simulink model "Architecture"  (R2020b)
settings: Solver=VariableStepAuto  StartTime=0.0  StopTime=10.0  RelTol=1e-3
undefined symbols (not defined in the file or in its folder): des, T
libraries: simulink x16
(part 4 of 6)

== system Architecture/PE11/Create Generator Selection Variable ==
  function : TriggerPort  TriggerType=function-call  VariantControl=(inherit)
  Repeating Sequence Stair : simulink/Sources/Repeating Sequence Stair  OutValues=[0 1].'  tsamp=-1  OutMin=[]  OutMax=[]  OutDataTypeStr=float('double')  OutputDataTypeScalingMode=Specify via dialog  OutDataType=float('double')  ConRadixGroup=Best Precision: Vector-wise  OutScaling=2^-12
  Out1 : Outport
  wires:
  Repeating Sequence Stair/1 -> Out1/1

== system Architecture/PE12/Create Generator Selection Variable ==
  function : TriggerPort  TriggerType=function-call  VariantControl=(inherit)
  Repeating Sequence Stair : simulink/Sources/Repeating Sequence Stair  OutValues=[0 1].'  tsamp=-1  OutMin=[]  OutMax=[]  OutDataTypeStr=float('double')  OutputDataTypeScalingMode=Specify via dialog  OutDataType=float('double')  ConRadixGroup=Best Precision: Vector-wise  OutScaling=2^-12
  Out1 : Outport
  wires:
  Repeating Sequence Stair/1 -> Out1/1

== system Architecture/PE13/Create Generator Selection Variable ==
  function : TriggerPort  TriggerType=function-call  VariantControl=(inherit)
  Repeating Sequence Stair : simulink/Sources/Repeating Sequence Stair  OutValues=[0 1].'  tsamp=-1  OutMin=[]  OutMax=[]  OutDataTypeStr=float('double')  OutputDataTypeScalingMode=Specify via dialog  OutDataType=float('double')  ConRadixGroup=Best Precision: Vector-wise  OutScaling=2^-12
  Out1 : Outport
  wires:
  Repeating Sequence Stair/1 -> Out1/1

== system Architecture/PE14/Create Generator Selection Variable ==
  function : TriggerPort  TriggerType=function-call  VariantControl=(inherit)
  Repeating Sequence Stair : simulink/Sources/Repeating Sequence Stair  OutValues=[0 1].'  tsamp=-1  OutMin=[]  OutMax=[]  OutDataTypeStr=float('double')  OutputDataTypeScalingMode=Specify via dialog  OutDataType=float('double')  ConRadixGroup=Best Precision: Vector-wise  OutScaling=2^-12
  Out1 : Outport
  wires:
  Repeating Sequence Stair/1 -> Out1/1

== system Architecture/PE15/Create Generator Selection Variable ==
  function : TriggerPort  TriggerType=function-call  VariantControl=(inherit)
  Repeating Sequence Stair : simulink/Sources/Repeating Sequence Stair  OutValues=[0 1].'  tsamp=-1  OutMin=[]  OutMax=[]  OutDataTypeStr=float('double')  OutputDataTypeScalingMode=Specify via dialog  OutDataType=float('double')  ConRadixGroup=Best Precision: Vector-wise  OutScaling=2^-12
  Out1 : Outport
  wires:
  Repeating Sequence Stair/1 -> Out1/1

== system Architecture/PE16/Create Generator Selection Variable ==
  function : TriggerPort  TriggerType=function-call  VariantControl=(inherit)
  Repeating Sequence Stair : simulink/Sources/Repeating Sequence Stair  OutValues=[0 1].'  tsamp=-1  OutMin=[]  OutMax=[]  OutDataTypeStr=float('double')  OutputDataTypeScalingMode=Specify via dialog  OutDataType=float('double')  ConRadixGroup=Best Precision: Vector-wise  OutScaling=2^-12
  Out1 : Outport
  wires:
  Repeating Sequence Stair/1 -> Out1/1

== system Architecture/PE2/Create Generator Selection Variable ==
  function : TriggerPort  TriggerType=function-call  VariantControl=(inherit)
  Repeating Sequence Stair : simulink/Sources/Repeating Sequence Stair  OutValues=[0 1].'  tsamp=-1  OutMin=[]  OutMax=[]  OutDataTypeStr=float('double')  OutputDataTypeScalingMode=Specify via dialog  OutDataType=float('double')  ConRadixGroup=Best Precision: Vector-wise  OutScaling=2^-12
  Out1 : Outport
  wires:
  Repeating Sequence Stair/1 -> Out1/1

== system Architecture/PE3/Create Generator Selection Variable ==
  function : TriggerPort  TriggerType=function-call  VariantControl=(inherit)
  Repeating Sequence Stair : simulink/Sources/Repeating Sequence Stair  OutValues=[0 1].'  tsamp=-1  OutMin=[]  OutMax=[]  OutDataTypeStr=float('double')  OutputDataTypeScalingMode=Specify via dialog  OutDataType=float('double')  ConRadixGroup=Best Precision: Vector-wise  OutScaling=2^-12
  Out1 : Outport
  wires:
  Repeating Sequence Stair/1 -> Out1/1

== system Architecture/PE4/Create Generator Selection Variable ==
  function : TriggerPort  TriggerType=function-call  VariantControl=(inherit)
  Repeating Sequence Stair : simulink/Sources/Repeating Sequence Stair  OutValues=[0 1].'  tsamp=-1  OutMin=[]  OutMax=[]  OutDataTypeStr=float('double')  OutputDataTypeScalingMode=Specify via dialog  OutDataType=float('double')  ConRadixGroup=Best Precision: Vector-wise  OutScaling=2^-12
  Out1 : Outport
  wires:
  Repeating Sequence Stair/1 -> Out1/1

== system Architecture/PE5/Create Generator Selection Variable ==
  function : TriggerPort  TriggerType=function-call  VariantControl=(inherit)
  Repeating Sequence Stair : simulink/Sources/Repeating Sequence Stair  OutValues=[0 1].'  tsamp=-1  OutMin=[]  OutMax=[]  OutDataTypeStr=float('double')  OutputDataTypeScalingMode=Specify via dialog  OutDataType=float('double')  ConRadixGroup=Best Precision: Vector-wise  OutScaling=2^-12
  Out1 : Outport
  wires:
  Repeating Sequence Stair/1 -> Out1/1

== system Architecture/PE6/Create Generator Selection Variable ==
  function : TriggerPort  TriggerType=function-call  VariantControl=(inherit)
  Repeating Sequence Stair : simulink/Sources/Repeating Sequence Stair  OutValues=[0 1].'  tsamp=-1  OutMin=[]  OutMax=[]  OutDataTypeStr=float('double')  OutputDataTypeScalingMode=Specify via dialog  OutDataType=float('double')  ConRadixGroup=Best Precision: Vector-wise  OutScaling=2^-12
  Out1 : Outport
  wires:
  Repeating Sequence Stair/1 -> Out1/1

== system Architecture/PE7/Create Generator Selection Variable ==
  function : TriggerPort  TriggerType=function-call  VariantControl=(inherit)
  Repeating Sequence Stair : simulink/Sources/Repeating Sequence Stair  OutValues=[0 1].'  tsamp=-1  OutMin=[]  OutMax=[]  OutDataTypeStr=float('double')  OutputDataTypeScalingMode=Specify via dialog  OutDataType=float('double')  ConRadixGroup=Best Precision: Vector-wise  OutScaling=2^-12
  Out1 : Outport
  wires:
  Repeating Sequence Stair/1 -> Out1/1

== system Architecture/PE8/Create Generator Selection Variable ==
  function : TriggerPort  TriggerType=function-call  VariantControl=(inherit)
  Repeating Sequence Stair : simulink/Sources/Repeating Sequence Stair  OutValues=[0 1].'  tsamp=-1  OutMin=[]  OutMax=[]  OutDataTypeStr=float('double')  OutputDataTypeScalingMode=Specify via dialog  OutDataType=float('double')  ConRadixGroup=Best Precision: Vector-wise  OutScaling=2^-12
  Out1 : Outport
  wires:
  Repeating Sequence Stair/1 -> Out1/1

== system Architecture/PE9/Create Generator Selection Variable ==
  function : TriggerPort  TriggerType=function-call  VariantControl=(inherit)
  Repeating Sequence Stair : simulink/Sources/Repeating Sequence Stair  OutValues=[0 1].'  tsamp=-1  OutMin=[]  OutMax=[]  OutDataTypeStr=float('double')  OutputDataTypeScalingMode=Specify via dialog  OutDataType=float('double')  ConRadixGroup=Best Precision: Vector-wise  OutScaling=2^-12
  Out1 : Outport
  wires:
  Repeating Sequence Stair/1 -> Out1/1

== system Architecture/Router1/Attribute Function ==
  MATLAB Function : MATLAB Function  TreatAsAtomicUnit=on
  __DMLF__EDE2FCE__ : EntityDepartureFunctionCallGenerator  TimingFunctionCallF1=Before entity departure  IsInsideAFB=on
  __DMLF__GA__ : GetAttribute  AttributeName=DST|ME  AttributeMissing=Error|Error  AttributeDefaultValue=1|1  AttributeTreatAsVector=1|1  AttributeSendTiming=Before entity departure|Before entity departure  EvaluatedDefaultAttributeValue={ [];[]}  IsInsideAFB=on
      settings: OutputPortMap=o1,o2
  __DMLF__SA__ : SetAttribute  AttributeName=RT  AttributeFrom=Signal port  EvaluatedAttributeValue={ []}  IsInsideAFB=on
  IN : PMIOPort  Side=Left
  OUT : PMIOPort  Port=2  Side=Right
  wires:
  MATLAB Function/1(out_RT) -> __DMLF__SA__/1
  __DMLF__GA__/2 -> MATLAB Function/2(ME)
  __DMLF__GA__/1 -> MATLAB Function/1(DST)
  __DMLF__EDE2FCE__/1 -> MATLAB Function/Trigger
  connections:
  __DMLF__SA__/RConn1 -- OUT/RConn1
  IN/RConn1 -- __DMLF__GA__/LConn1
  __DMLF__GA__/RConn1 -- __DMLF__EDE2FCE__/LConn1
  __DMLF__SA__/LConn1 -- __DMLF__EDE2FCE__/RConn1

== system Architecture/Router1/Clocked FIFO1 ==
  Event-Based Random Number : EventBasedRandomNumber  Distribution=Gaussian (normal)  meanNorm=E  stdNorm=S
  FIFO Queue : FIFOQueue  Capacity=F  StatNumberInBlock=on
      settings: OutputPortMap=o1
  Release Gate : ReleaseGate  OpenGateUpon=Function call from port fcn
  Time-Based Function-Call Generator : TimeBasedFunctionCallGenerator  EventGenerationMode=Period from port  Period=T
  Input : PMIOPort  Side=Left
  Output : PMIOPort  Port=2  Side=Right
  #n : Outport
  wires:
  Event-Based Random Number/1 -> Time-Based Function-Call Generator/1
  FIFO Queue/1 -> #n/1
  Time-Based Function-Call Generator/1 -> Release Gate/1
  connections:
  FIFO Queue/RConn1 -- Release Gate/LConn1
  Release Gate/RConn1 -- Output/RConn1
  FIFO Queue/LConn1 -- Input/RConn1

== system Architecture/Router1/Clocked FIFO2 ==
  Event-Based Random Number : EventBasedRandomNumber  Distribution=Gaussian (normal)  meanNorm=E  stdNorm=S
  FIFO Queue : FIFOQueue  Capacity=F  StatNumberInBlock=on
      settings: OutputPortMap=o1
  Release Gate : ReleaseGate  OpenGateUpon=Function call from port fcn
  Time-Based Function-Call Generator : TimeBasedFunctionCallGenerator  EventGenerationMode=Period from port  Period=T
  Input : PMIOPort  Side=Left
  Output : PMIOPort  Port=2  Side=Right
  #n : Outport
  wires:
  Event-Based Random Number/1 -> Time-Based Function-Call Generator/1
  FIFO Queue/1 -> #n/1
  Time-Based Function-Call Generator/1 -> Release Gate/1
  connections:
  FIFO Queue/RConn1 -- Release Gate/LConn1
  Release Gate/RConn1 -- Output/RConn1
  FIFO Queue/LConn1 -- Input/RConn1

== system Architecture/Router1/Clocked FIFO3 ==
  Event-Based Random Number : EventBasedRandomNumber  Distribution=Gaussian (normal)  meanNorm=E  stdNorm=S
  FIFO Queue : FIFOQueue  Capacity=F  StatNumberInBlock=on
      settings: OutputPortMap=o1
  Release Gate : ReleaseGate  OpenGateUpon=Function call from port fcn
  Time-Based Function-Call Generator : TimeBasedFunctionCallGenerator  EventGenerationMode=Period from port  Period=T
  Input : PMIOPort  Side=Left
  Output : PMIOPort  Port=2  Side=Right
  #n : Outport
  wires:
  Event-Based Random Number/1 -> Time-Based Function-Call Generator/1
  FIFO Queue/1 -> #n/1
  Time-Based Function-Call Generator/1 -> Release Gate/1
  connections:
  FIFO Queue/RConn1 -- Release Gate/LConn1
  Release Gate/RConn1 -- Output/RConn1
  FIFO Queue/LConn1 -- Input/RConn1

== system Architecture/Router1/Clocked FIFO4 ==
  Event-Based Random Number : EventBasedRandomNumber  Distribution=Gaussian (normal)  meanNorm=E  stdNorm=S
  FIFO Queue : FIFOQueue  Capacity=F  StatNumberInBlock=on
      settings: OutputPortMap=o1
  Release Gate : ReleaseGate  OpenGateUpon=Function call from port fcn
  Time-Based Function-Call Generator : TimeBasedFunctionCallGenerator  EventGenerationMode=Period from port  Period=T
  Input : PMIOPort  Side=Left
  Output : PMIOPort  Port=2  Side=Right
  #n : Outport
  wires:
  Event-Based Random Number/1 -> Time-Based Function-Call Generator/1
  FIFO Queue/1 -> #n/1
  Time-Based Function-Call Generator/1 -> Release Gate/1
  connections:
  FIFO Queue/RConn1 -- Release Gate/LConn1
  Release Gate/RConn1 -- Output/RConn1
  FIFO Queue/LConn1 -- Input/RConn1

== system Architecture/Router1/Clocked FIFO5 ==
  Event-Based Random Number : EventBasedRandomNumber  Distribution=Gaussian (normal)  meanNorm=E  stdNorm=S
  FIFO Queue : FIFOQueue  Capacity=F  StatNumberInBlock=on
      settings: OutputPortMap=o1
  Release Gate : ReleaseGate  OpenGateUpon=Function call from port fcn
  Time-Based Function-Call Generator : TimeBasedFunctionCallGenerator  EventGenerationMode=Period from port  Period=T
  Input : PMIOPort  Side=Left
  Output : PMIOPort  Port=2  Side=Right
  #n : Outport
  wires:
  Event-Based Random Number/1 -> Time-Based Function-Call Generator/1
  FIFO Queue/1 -> #n/1
  Time-Based Function-Call Generator/1 -> Release Gate/1
  connections:
  FIFO Queue/RConn1 -- Release Gate/LConn1
  Release Gate/RConn1 -- Output/RConn1
  FIFO Queue/LConn1 -- Input/RConn1

== system Architecture/Router10/Attribute Function ==
  MATLAB Function : MATLAB Function  TreatAsAtomicUnit=on
  __DMLF__EDE2FCE__ : EntityDepartureFunctionCallGenerator  TimingFunctionCallF1=Before entity departure  IsInsideAFB=on
  __DMLF__GA__ : GetAttribute  AttributeName=DST|ME  AttributeMissing=Error|Error  AttributeDefaultValue=1|1  AttributeTreatAsVector=1|1  AttributeSendTiming=Before entity departure|Before entity departure  EvaluatedDefaultAttributeValue={ [];[]}  IsInsideAFB=on
      settings: OutputPortMap=o1,o2
  __DMLF__SA__ : SetAttribute  AttributeName=RT  AttributeFrom=Signal port  EvaluatedAttributeValue={ []}  IsInsideAFB=on
  IN : PMIOPort  Side=Left
  OUT : PMIOPort  Port=2  Side=Right
  wires:
  MATLAB Function/1(out_RT) -> __DMLF__SA__/1
  __DMLF__GA__/2 -> MATLAB Function/2(ME)
  __DMLF__GA__/1 -> MATLAB Function/1(DST)
  __DMLF__EDE2FCE__/1 -> MATLAB Function/Trigger
  connections:
  __DMLF__SA__/RConn1 -- OUT/RConn1
  IN/RConn1 -- __DMLF__GA__/LConn1
  __DMLF__GA__/RConn1 -- __DMLF__EDE2FCE__/LConn1
  __DMLF__SA__/LConn1 -- __DMLF__EDE2FCE__/RConn1

== system Architecture/Router10/Clocked FIFO1 ==
  Event-Based Random Number : EventBasedRandomNumber  Distribution=Gaussian (normal)  meanNorm=E  stdNorm=S
  FIFO Queue : FIFOQueue  Capacity=F  StatNumberInBlock=on
      settings: OutputPortMap=o1
  Release Gate : ReleaseGate  OpenGateUpon=Function call from port fcn
  Time-Based Function-Call Generator : TimeBasedFunctionCallGenerator  EventGenerationMode=Period from port  Period=T
  Input : PMIOPort  Side=Left
  Output : PMIOPort  Port=2  Side=Right
  #n : Outport
  wires:
  Event-Based Random Number/1 -> Time-Based Function-Call Generator/1
  FIFO Queue/1 -> #n/1
  Time-Based Function-Call Generator/1 -> Release Gate/1
  connections:
  FIFO Queue/RConn1 -- Release Gate/LConn1
  Release Gate/RConn1 -- Output/RConn1
  FIFO Queue/LConn1 -- Input/RConn1

== system Architecture/Router10/Clocked FIFO2 ==
  Event-Based Random Number : EventBasedRandomNumber  Distribution=Gaussian (normal)  meanNorm=E  stdNorm=S
  FIFO Queue : FIFOQueue  Capacity=F  StatNumberInBlock=on
      settings: OutputPortMap=o1
  Release Gate : ReleaseGate  OpenGateUpon=Function call from port fcn
  Time-Based Function-Call Generator : TimeBasedFunctionCallGenerator  EventGenerationMode=Period from port  Period=T
  Input : PMIOPort  Side=Left
  Output : PMIOPort  Port=2  Side=Right
  #n : Outport
  wires:
  Event-Based Random Number/1 -> Time-Based Function-Call Generator/1
  FIFO Queue/1 -> #n/1
  Time-Based Function-Call Generator/1 -> Release Gate/1
  connections:
  FIFO Queue/RConn1 -- Release Gate/LConn1
  Release Gate/RConn1 -- Output/RConn1
  FIFO Queue/LConn1 -- Input/RConn1

== system Architecture/Router10/Clocked FIFO3 ==
  Event-Based Random Number : EventBasedRandomNumber  Distribution=Gaussian (normal)  meanNorm=E  stdNorm=S
  FIFO Queue : FIFOQueue  Capacity=F  StatNumberInBlock=on
      settings: OutputPortMap=o1
  Release Gate : ReleaseGate  OpenGateUpon=Function call from port fcn
  Time-Based Function-Call Generator : TimeBasedFunctionCallGenerator  EventGenerationMode=Period from port  Period=T
  Input : PMIOPort  Side=Left
  Output : PMIOPort  Port=2  Side=Right
  #n : Outport
  wires:
  Event-Based Random Number/1 -> Time-Based Function-Call Generator/1
  FIFO Queue/1 -> #n/1
  Time-Based Function-Call Generator/1 -> Release Gate/1
  connections:
  FIFO Queue/RConn1 -- Release Gate/LConn1
  Release Gate/RConn1 -- Output/RConn1
  FIFO Queue/LConn1 -- Input/RConn1

== system Architecture/Router10/Clocked FIFO4 ==
  Event-Based Random Number : EventBasedRandomNumber  Distribution=Gaussian (normal)  meanNorm=E  stdNorm=S
  FIFO Queue : FIFOQueue  Capacity=F  StatNumberInBlock=on
      settings: OutputPortMap=o1
  Release Gate : ReleaseGate  OpenGateUpon=Function call from port fcn
  Time-Based Function-Call Generator : TimeBasedFunctionCallGenerator  EventGenerationMode=Period from port  Period=T
  Input : PMIOPort  Side=Left
  Output : PMIOPort  Port=2  Side=Right
  #n : Outport
  wires:
  Event-Based Random Number/1 -> Time-Based Function-Call Generator/1
  FIFO Queue/1 -> #n/1
  Time-Based Function-Call Generator/1 -> Release Gate/1
  connections:
  FIFO Queue/RConn1 -- Release Gate/LConn1
  Release Gate/RConn1 -- Output/RConn1
  FIFO Queue/LConn1 -- Input/RConn1

== system Architecture/Router10/Clocked FIFO5 ==
  Event-Based Random Number : EventBasedRandomNumber  Distribution=Gaussian (normal)  meanNorm=E  stdNorm=S
  FIFO Queue : FIFOQueue  Capacity=F  StatNumberInBlock=on
      settings: OutputPortMap=o1
  Release Gate : ReleaseGate  OpenGateUpon=Function call from port fcn
  Time-Based Function-Call Generator : TimeBasedFunctionCallGenerator  EventGenerationMode=Period from port  Period=T
  Input : PMIOPort  Side=Left
  Output : PMIOPort  Port=2  Side=Right
  #n : Outport
  wires:
  Event-Based Random Number/1 -> Time-Based Function-Call Generator/1
  FIFO Queue/1 -> #n/1
  Time-Based Function-Call Generator/1 -> Release Gate/1
  connections:
  FIFO Queue/RConn1 -- Release Gate/LConn1
  Release Gate/RConn1 -- Output/RConn1
  FIFO Queue/LConn1 -- Input/RConn1

== system Architecture/Router11/Attribute Function ==
  MATLAB Function : MATLAB Function  TreatAsAtomicUnit=on
  __DMLF__EDE2FCE__ : EntityDepartureFunctionCallGenerator  TimingFunctionCallF1=Before entity departure  IsInsideAFB=on
  __DMLF__GA__ : GetAttribute  AttributeName=DST|ME  AttributeMissing=Error|Error  AttributeDefaultValue=1|1  AttributeTreatAsVector=1|1  AttributeSendTiming=Before entity departure|Before entity departure  EvaluatedDefaultAttributeValue={ [];[]}  IsInsideAFB=on
      settings: OutputPortMap=o1,o2
  __DMLF__SA__ : SetAttribute  AttributeName=RT  AttributeFrom=Signal port  EvaluatedAttributeValue={ []}  IsInsideAFB=on
  IN : PMIOPort  Side=Left
  OUT : PMIOPort  Port=2  Side=Right
  wires:
  MATLAB Function/1(out_RT) -> __DMLF__SA__/1
  __DMLF__GA__/2 -> MATLAB Function/2(ME)
  __DMLF__GA__/1 -> MATLAB Function/1(DST)
  __DMLF__EDE2FCE__/1 -> MATLAB Function/Trigger
  connections:
  __DMLF__SA__/RConn1 -- OUT/RConn1
  IN/RConn1 -- __DMLF__GA__/LConn1
  __DMLF__GA__/RConn1 -- __DMLF__EDE2FCE__/LConn1
  __DMLF__SA__/LConn1 -- __DMLF__EDE2FCE__/RConn1

== system Architecture/Router11/Clocked FIFO1 ==
  Event-Based Random Number : EventBasedRandomNumber  Distribution=Gaussian (normal)  meanNorm=E  stdNorm=S
  FIFO Queue : FIFOQueue  Capacity=F  StatNumberInBlock=on
      settings: OutputPortMap=o1
  Release Gate : ReleaseGate  OpenGateUpon=Function call from port fcn
  Time-Based Function-Call Generator : TimeBasedFunctionCallGenerator  EventGenerationMode=Period from port  Period=T
  Input : PMIOPort  Side=Left
  Output : PMIOPort  Port=2  Side=Right
  #n : Outport
  wires:
  Event-Based Random Number/1 -> Time-Based Function-Call Generator/1
  FIFO Queue/1 -> #n/1
  Time-Based Function-Call Generator/1 -> Release Gate/1
  connections:
  FIFO Queue/RConn1 -- Release Gate/LConn1
  Release Gate/RConn1 -- Output/RConn1
  FIFO Queue/LConn1 -- Input/RConn1

== system Architecture/Router11/Clocked FIFO2 ==
  Event-Based Random Number : EventBasedRandomNumber  Distribution=Gaussian (normal)  meanNorm=E  stdNorm=S
  FIFO Queue : FIFOQueue  Capacity=F  StatNumberInBlock=on
      settings: OutputPortMap=o1
  Release Gate : ReleaseGate  OpenGateUpon=Function call from port fcn
  Time-Based Function-Call Generator : TimeBasedFunctionCallGenerator  EventGenerationMode=Period from port  Period=T
  Input : PMIOPort  Side=Left
  Output : PMIOPort  Port=2  Side=Right
  #n : Outport
  wires:
  Event-Based Random Number/1 -> Time-Based Function-Call Generator/1
  FIFO Queue/1 -> #n/1
  Time-Based Function-Call Generator/1 -> Release Gate/1
  connections:
  FIFO Queue/RConn1 -- Release Gate/LConn1
  Release Gate/RConn1 -- Output/RConn1
  FIFO Queue/LConn1 -- Input/RConn1

== system Architecture/Router11/Clocked FIFO3 ==
  Event-Based Random Number : EventBasedRandomNumber  Distribution=Gaussian (normal)  meanNorm=E  stdNorm=S
  FIFO Queue : FIFOQueue  Capacity=F  StatNumberInBlock=on
      settings: OutputPortMap=o1
  Release Gate : ReleaseGate  OpenGateUpon=Function call from port fcn
  Time-Based Function-Call Generator : TimeBasedFunctionCallGenerator  EventGenerationMode=Period from port  Period=T
  Input : PMIOPort  Side=Left
  Output : PMIOPort  Port=2  Side=Right
  #n : Outport
  wires:
  Event-Based Random Number/1 -> Time-Based Function-Call Generator/1
  FIFO Queue/1 -> #n/1
  Time-Based Function-Call Generator/1 -> Release Gate/1
  connections:
  FIFO Queue/RConn1 -- Release Gate/LConn1
  Release Gate/RConn1 -- Output/RConn1
  FIFO Queue/LConn1 -- Input/RConn1

== system Architecture/Router11/Clocked FIFO4 ==
  Event-Based Random Number : EventBasedRandomNumber  Distribution=Gaussian (normal)  meanNorm=E  stdNorm=S
  FIFO Queue : FIFOQueue  Capacity=F  StatNumberInBlock=on
      settings: OutputPortMap=o1
  Release Gate : ReleaseGate  OpenGateUpon=Function call from port fcn
  Time-Based Function-Call Generator : TimeBasedFunctionCallGenerator  EventGenerationMode=Period from port  Period=T
  Input : PMIOPort  Side=Left
  Output : PMIOPort  Port=2  Side=Right
  #n : Outport
  wires:
  Event-Based Random Number/1 -> Time-Based Function-Call Generator/1
  FIFO Queue/1 -> #n/1
  Time-Based Function-Call Generator/1 -> Release Gate/1
  connections:
  FIFO Queue/RConn1 -- Release Gate/LConn1
  Release Gate/RConn1 -- Output/RConn1
  FIFO Queue/LConn1 -- Input/RConn1

== system Architecture/Router11/Clocked FIFO5 ==
  Event-Based Random Number : EventBasedRandomNumber  Distribution=Gaussian (normal)  meanNorm=E  stdNorm=S
  FIFO Queue : FIFOQueue  Capacity=F  StatNumberInBlock=on
      settings: OutputPortMap=o1
  Release Gate : ReleaseGate  OpenGateUpon=Function call from port fcn
  Time-Based Function-Call Generator : TimeBasedFunctionCallGenerator  EventGenerationMode=Period from port  Period=T
  Input : PMIOPort  Side=Left
  Output : PMIOPort  Port=2  Side=Right
  #n : Outport
  wires:
  Event-Based Random Number/1 -> Time-Based Function-Call Generator/1
  FIFO Queue/1 -> #n/1
  Time-Based Function-Call Generator/1 -> Release Gate/1
  connections:
  FIFO Queue/RConn1 -- Release Gate/LConn1
  Release Gate/RConn1 -- Output/RConn1
  FIFO Queue/LConn1 -- Input/RConn1

== system Architecture/Router12/Attribute Function ==
  MATLAB Function : MATLAB Function  TreatAsAtomicUnit=on
  __DMLF__EDE2FCE__ : EntityDepartureFunctionCallGenerator  TimingFunctionCallF1=Before entity departure  IsInsideAFB=on
  __DMLF__GA__ : GetAttribute  AttributeName=DST|ME  AttributeMissing=Error|Error  AttributeDefaultValue=1|1  AttributeTreatAsVector=1|1  AttributeSendTiming=Before entity departure|Before entity departure  EvaluatedDefaultAttributeValue={ [];[]}  IsInsideAFB=on
      settings: OutputPortMap=o1,o2
  __DMLF__SA__ : SetAttribute  AttributeName=RT  AttributeFrom=Signal port  EvaluatedAttributeValue={ []}  IsInsideAFB=on
  IN : PMIOPort  Side=Left
  OUT : PMIOPort  Port=2  Side=Right
  wires:
  MATLAB Function/1(out_RT) -> __DMLF__SA__/1
  __DMLF__GA__/2 -> MATLAB Function/2(ME)
  __DMLF__GA__/1 -> MATLAB Function/1(DST)
  __DMLF__EDE2FCE__/1 -> MATLAB Function/Trigger
  connections:
  __DMLF__SA__/RConn1 -- OUT/RConn1
  IN/RConn1 -- __DMLF__GA__/LConn1
  __DMLF__GA__/RConn1 -- __DMLF__EDE2FCE__/LConn1
  __DMLF__SA__/LConn1 -- __DMLF__EDE2FCE__/RConn1

== system Architecture/Router12/Clocked FIFO1 ==
  Event-Based Random Number : EventBasedRandomNumber  Distribution=Gaussian (normal)  meanNorm=E  stdNorm=S
  FIFO Queue : FIFOQueue  Capacity=F  StatNumberInBlock=on
      settings: OutputPortMap=o1
  Release Gate : ReleaseGate  OpenGateUpon=Function call from port fcn
  Time-Based Function-Call Generator : TimeBasedFunctionCallGenerator  EventGenerationMode=Period from port  Period=T
  Input : PMIOPort  Side=Left
  Output : PMIOPort  Port=2  Side=Right
  #n : Outport
  wires:
  Event-Based Random Number/1 -> Time-Based Function-Call Generator/1
  FIFO Queue/1 -> #n/1
  Time-Based Function-Call Generator/1 -> Release Gate/1
  connections:
  FIFO Queue/RConn1 -- Release Gate/LConn1
  Release Gate/RConn1 -- Output/RConn1
  FIFO Queue/LConn1 -- Input/RConn1

== system Architecture/Router12/Clocked FIFO2 ==
  Event-Based Random Number : EventBasedRandomNumber  Distribution=Gaussian (normal)  meanNorm=E  stdNorm=S
  FIFO Queue : FIFOQueue  Capacity=F  StatNumberInBlock=on
      settings: OutputPortMap=o1
  Release Gate : ReleaseGate  OpenGateUpon=Function call from port fcn
  Time-Based Function-Call Generator : TimeBasedFunctionCallGenerator  EventGenerationMode=Period from port  Period=T
  Input : PMIOPort  Side=Left
  Output : PMIOPort  Port=2  Side=Right
  #n : Outport
  wires:
  Event-Based Random Number/1 -> Time-Based Function-Call Generator/1
  FIFO Queue/1 -> #n/1
  Time-Based Function-Call Generator/1 -> Release Gate/1
  connections:
  FIFO Queue/RConn1 -- Release Gate/LConn1
  Release Gate/RConn1 -- Output/RConn1
  FIFO Queue/LConn1 -- Input/RConn1

== system Architecture/Router12/Clocked FIFO3 ==
  Event-Based Random Number : EventBasedRandomNumber  Distribution=Gaussian (normal)  meanNorm=E  stdNorm=S
  FIFO Queue : FIFOQueue  Capacity=F  StatNumberInBlock=on
      settings: OutputPortMap=o1
  Release Gate : ReleaseGate  OpenGateUpon=Function call from port fcn
  Time-Based Function-Call Generator : TimeBasedFunctionCallGenerator  EventGenerationMode=Period from port  Period=T
  Input : PMIOPort  Side=Left
  Output : PMIOPort  Port=2  Side=Right
  #n : Outport
  wires:
  Event-Based Random Number/1 -> Time-Based Function-Call Generator/1
  FIFO Queue/1 -> #n/1
  Time-Based Function-Call Generator/1 -> Release Gate/1
  connections:
  FIFO Queue/RConn1 -- Release Gate/LConn1
  Release Gate/RConn1 -- Output/RConn1
  FIFO Queue/LConn1 -- Input/RConn1

== system Architecture/Router12/Clocked FIFO4 ==
  Event-Based Random Number : EventBasedRandomNumber  Distribution=Gaussian (normal)  meanNorm=E  stdNorm=S
  FIFO Queue : FIFOQueue  Capacity=F  StatNumberInBlock=on
      settings: OutputPortMap=o1
  Release Gate : ReleaseGate  OpenGateUpon=Function call from port fcn
  Time-Based Function-Call Generator : TimeBasedFunctionCallGenerator  EventGenerationMode=Period from port  Period=T
  Input : PMIOPort  Side=Left
  Output : PMIOPort  Port=2  Side=Right
  #n : Outport
  wires:
  Event-Based Random Number/1 -> Time-Based Function-Call Generator/1
  FIFO Queue/1 -> #n/1
  Time-Based Function-Call Generator/1 -> Release Gate/1
  connections:
  FIFO Queue/RConn1 -- Release Gate/LConn1
  Release Gate/RConn1 -- Output/RConn1
  FIFO Queue/LConn1 -- Input/RConn1

== system Architecture/Router12/Clocked FIFO5 ==
  Event-Based Random Number : EventBasedRandomNumber  Distribution=Gaussian (normal)  meanNorm=E  stdNorm=S
  FIFO Queue : FIFOQueue  Capacity=F  StatNumberInBlock=on
      settings: OutputPortMap=o1
  Release Gate : ReleaseGate  OpenGateUpon=Function call from port fcn
  Time-Based Function-Call Generator : TimeBasedFunctionCallGenerator  EventGenerationMode=Period from port  Period=T
  Input : PMIOPort  Side=Left
  Output : PMIOPort  Port=2  Side=Right
  #n : Outport
  wires:
  Event-Based Random Number/1 -> Time-Based Function-Call Generator/1
  FIFO Queue/1 -> #n/1
  Time-Based Function-Call Generator/1 -> Release Gate/1
  connections:
  FIFO Queue/RConn1 -- Release Gate/LConn1
  Release Gate/RConn1 -- Output/RConn1
  FIFO Queue/LConn1 -- Input/RConn1

== system Architecture/Router13/Attribute Function ==
  MATLAB Function : MATLAB Function  TreatAsAtomicUnit=on
  __DMLF__EDE2FCE__ : EntityDepartureFunctionCallGenerator  TimingFunctionCallF1=Before entity departure  IsInsideAFB=on
  __DMLF__GA__ : GetAttribute  AttributeName=DST|ME  AttributeMissing=Error|Error  AttributeDefaultValue=1|1  AttributeTreatAsVector=1|1  AttributeSendTiming=Before entity departure|Before entity departure  EvaluatedDefaultAttributeValue={ [];[]}  IsInsideAFB=on
      settings: OutputPortMap=o1,o2
  __DMLF__SA__ : SetAttribute  AttributeName=RT  AttributeFrom=Signal port  EvaluatedAttributeValue={ []}  IsInsideAFB=on
  IN : PMIOPort  Side=Left
  OUT : PMIOPort  Port=2  Side=Right
  wires:
  MATLAB Function/1(out_RT) -> __DMLF__SA__/1
  __DMLF__GA__/2 -> MATLAB Function/2(ME)
  __DMLF__GA__/1 -> MATLAB Function/1(DST)
  __DMLF__EDE2FCE__/1 -> MATLAB Function/Trigger
  connections:
  __DMLF__SA__/RConn1 -- OUT/RConn1
  IN/RConn1 -- __DMLF__GA__/LConn1
  __DMLF__GA__/RConn1 -- __DMLF__EDE2FCE__/LConn1
  __DMLF__SA__/LConn1 -- __DMLF__EDE2FCE__/RConn1

== system Architecture/Router13/Clocked FIFO1 ==
  Event-Based Random Number : EventBasedRandomNumber  Distribution=Gaussian (normal)  meanNorm=E  stdNorm=S
  FIFO Queue : FIFOQueue  Capacity=F  StatNumberInBlock=on
      settings: OutputPortMap=o1
  Release Gate : ReleaseGate  OpenGateUpon=Function call from port fcn
  Time-Based Function-Call Generator : TimeBasedFunctionCallGenerator  EventGenerationMode=Period from port  Period=T
  Input : PMIOPort  Side=Left
  Output : PMIOPort  Port=2  Side=Right
  #n : Outport
  wires:
  Event-Based Random Number/1 -> Time-Based Function-Call Generator/1
  FIFO Queue/1 -> #n/1
  Time-Based Function-Call Generator/1 -> Release Gate/1
  connections:
  FIFO Queue/RConn1 -- Release Gate/LConn1
  Release Gate/RConn1 -- Output/RConn1
  FIFO Queue/LConn1 -- Input/RConn1

== system Architecture/Router13/Clocked FIFO2 ==
  Event-Based Random Number : EventBasedRandomNumber  Distribution=Gaussian (normal)  meanNorm=E  stdNorm=S
  FIFO Queue : FIFOQueue  Capacity=F  StatNumberInBlock=on
      settings: OutputPortMap=o1
  Release Gate : ReleaseGate  OpenGateUpon=Function call from port fcn
  Time-Based Function-Call Generator : TimeBasedFunctionCallGenerator  EventGenerationMode=Period from port  Period=T
  Input : PMIOPort  Side=Left
  Output : PMIOPort  Port=2  Side=Right
  #n : Outport
  wires:
  Event-Based Random Number/1 -> Time-Based Function-Call Generator/1
  FIFO Queue/1 -> #n/1
  Time-Based Function-Call Generator/1 -> Release Gate/1
  connections:
  FIFO Queue/RConn1 -- Release Gate/LConn1
  Release Gate/RConn1 -- Output/RConn1
  FIFO Queue/LConn1 -- Input/RConn1

== system Architecture/Router13/Clocked FIFO3 ==
  Event-Based Random Number : EventBasedRandomNumber  Distribution=Gaussian (normal)  meanNorm=E  stdNorm=S
  FIFO Queue : FIFOQueue  Capacity=F  StatNumberInBlock=on
      settings: OutputPortMap=o1
  Release Gate : ReleaseGate  OpenGateUpon=Function call from port fcn
  Time-Based Function-Call Generator : TimeBasedFunctionCallGenerator  EventGenerationMode=Period from port  Period=T
  Input : PMIOPort  Side=Left
  Output : PMIOPort  Port=2  Side=Right
  #n : Outport
  wires:
  Event-Based Random Number/1 -> Time-Based Function-Call Generator/1
  FIFO Queue/1 -> #n/1
  Time-Based Function-Call Generator/1 -> Release Gate/1
  connections:
  FIFO Queue/RConn1 -- Release Gate/LConn1
  Release Gate/RConn1 -- Output/RConn1
  FIFO Queue/LConn1 -- Input/RConn1

== system Architecture/Router13/Clocked FIFO4 ==
  Event-Based Random Number : EventBasedRandomNumber  Distribution=Gaussian (normal)  meanNorm=E  stdNorm=S
  FIFO Queue : FIFOQueue  Capacity=F  StatNumberInBlock=on
      settings: OutputPortMap=o1
  Release Gate : ReleaseGate  OpenGateUpon=Function call from port fcn
  Time-Based Function-Call Generator : TimeBasedFunctionCallGenerator  EventGenerationMode=Period from port  Period=T
  Input : PMIOPort  Side=Left
  Output : PMIOPort  Port=2  Side=Right
  #n : Outport
  wires:
  Event-Based Random Number/1 -> Time-Based Function-Call Generator/1
  FIFO Queue/1 -> #n/1
  Time-Based Function-Call Generator/1 -> Release Gate/1
  connections:
  FIFO Queue/RConn1 -- Release Gate/LConn1
  Release Gate/RConn1 -- Output/RConn1
  FIFO Queue/LConn1 -- Input/RConn1

== system Architecture/Router13/Clocked FIFO5 ==
  Event-Based Random Number : EventBasedRandomNumber  Distribution=Gaussian (normal)  meanNorm=E  stdNorm=S
  FIFO Queue : FIFOQueue  Capacity=F  StatNumberInBlock=on
      settings: OutputPortMap=o1
  Release Gate : ReleaseGate  OpenGateUpon=Function call from port fcn
  Time-Based Function-Call Generator : TimeBasedFunctionCallGenerator  EventGenerationMode=Period from port  Period=T
  Input : PMIOPort  Side=Left
  Output : PMIOPort  Port=2  Side=Right
  #n : Outport
  wires:
  Event-Based Random Number/1 -> Time-Based Function-Call Generator/1
  FIFO Queue/1 -> #n/1
  Time-Based Function-Call Generator/1 -> Release Gate/1
  connections:
  FIFO Queue/RConn1 -- Release Gate/LConn1
  Release Gate/RConn1 -- Output/RConn1
  FIFO Queue/LConn1 -- Input/RConn1

== system Architecture/Router14/Attribute Function ==
  MATLAB Function : MATLAB Function  TreatAsAtomicUnit=on
  __DMLF__EDE2FCE__ : EntityDepartureFunctionCallGenerator  TimingFunctionCallF1=Before entity departure  IsInsideAFB=on
  __DMLF__GA__ : GetAttribute  AttributeName=DST|ME  AttributeMissing=Error|Error  AttributeDefaultValue=1|1  AttributeTreatAsVector=1|1  AttributeSendTiming=Before entity departure|Before entity departure  EvaluatedDefaultAttributeValue={ [];[]}  IsInsideAFB=on
      settings: OutputPortMap=o1,o2
  __DMLF__SA__ : SetAttribute  AttributeName=RT  AttributeFrom=Signal port  EvaluatedAttributeValue={ []}  IsInsideAFB=on
  IN : PMIOPort  Side=Left
  OUT : PMIOPort  Port=2  Side=Right
  wires:
  MATLAB Function/1(out_RT) -> __DMLF__SA__/1
  __DMLF__GA__/2 -> MATLAB Function/2(ME)
  __DMLF__GA__/1 -> MATLAB Function/1(DST)
  __DMLF__EDE2FCE__/1 -> MATLAB Function/Trigger
  connections:
  __DMLF__SA__/RConn1 -- OUT/RConn1
  IN/RConn1 -- __DMLF__GA__/LConn1
  __DMLF__GA__/RConn1 -- __DMLF__EDE2FCE__/LConn1
  __DMLF__SA__/LConn1 -- __DMLF__EDE2FCE__/RConn1

== system Architecture/Router14/Clocked FIFO1 ==
  Event-Based Random Number : EventBasedRandomNumber  Distribution=Gaussian (normal)  meanNorm=E  stdNorm=S
  FIFO Queue : FIFOQueue  Capacity=F  StatNumberInBlock=on
      settings: OutputPortMap=o1
  Release Gate : ReleaseGate  OpenGateUpon=Function call from port fcn
  Time-Based Function-Call Generator : TimeBasedFunctionCallGenerator  EventGenerationMode=Period from port  Period=T
  Input : PMIOPort  Side=Left
  Output : PMIOPort  Port=2  Side=Right
  #n : Outport
  wires:
  Event-Based Random Number/1 -> Time-Based Function-Call Generator/1
  FIFO Queue/1 -> #n/1
  Time-Based Function-Call Generator/1 -> Release Gate/1
  connections:
  FIFO Queue/RConn1 -- Release Gate/LConn1
  Release Gate/RConn1 -- Output/RConn1
  FIFO Queue/LConn1 -- Input/RConn1

== system Architecture/Router14/Clocked FIFO2 ==
  Event-Based Random Number : EventBasedRandomNumber  Distribution=Gaussian (normal)  meanNorm=E  stdNorm=S
  FIFO Queue : FIFOQueue  Capacity=F  StatNumberInBlock=on
      settings: OutputPortMap=o1
  Release Gate : ReleaseGate  OpenGateUpon=Function call from port fcn
  Time-Based Function-Call Generator : TimeBasedFunctionCallGenerator  EventGenerationMode=Period from port  Period=T
  Input : PMIOPort  Side=Left
  Output : PMIOPort  Port=2  Side=Right
  #n : Outport
  wires:
  Event-Based Random Number/1 -> Time-Based Function-Call Generator/1
  FIFO Queue/1 -> #n/1
  Time-Based Function-Call Generator/1 -> Release Gate/1
  connections:
  FIFO Queue/RConn1 -- Release Gate/LConn1
  Release Gate/RConn1 -- Output/RConn1
  FIFO Queue/LConn1 -- Input/RConn1

== system Architecture/Router14/Clocked FIFO3 ==
  Event-Based Random Number : EventBasedRandomNumber  Distribution=Gaussian (normal)  meanNorm=E  stdNorm=S
  FIFO Queue : FIFOQueue  Capacity=F  StatNumberInBlock=on
      settings: OutputPortMap=o1
  Release Gate : ReleaseGate  OpenGateUpon=Function call from port fcn
  Time-Based Function-Call Generator : TimeBasedFunctionCallGenerator  EventGenerationMode=Period from port  Period=T
  Input : PMIOPort  Side=Left
  Output : PMIOPort  Port=2  Side=Right
  #n : Outport
  wires:
  Event-Based Random Number/1 -> Time-Based Function-Call Generator/1
  FIFO Queue/1 -> #n/1
  Time-Based Function-Call Generator/1 -> Release Gate/1
  connections:
  FIFO Queue/RConn1 -- Release Gate/LConn1
  Release Gate/RConn1 -- Output/RConn1
  FIFO Queue/LConn1 -- Input/RConn1

== system Architecture/Router14/Clocked FIFO4 ==
  Event-Based Random Number : EventBasedRandomNumber  Distribution=Gaussian (normal)  meanNorm=E  stdNorm=S
  FIFO Queue : FIFOQueue  Capacity=F  StatNumberInBlock=on
      settings: OutputPortMap=o1
  Release Gate : ReleaseGate  OpenGateUpon=Function call from port fcn
  Time-Based Function-Call Generator : TimeBasedFunctionCallGenerator  EventGenerationMode=Period from port  Period=T
  Input : PMIOPort  Side=Left
  Output : PMIOPort  Port=2  Side=Right
  #n : Outport
  wires:
  Event-Based Random Number/1 -> Time-Based Function-Call Generator/1
  FIFO Queue/1 -> #n/1
  Time-Based Function-Call Generator/1 -> Release Gate/1
  connections:
  FIFO Queue/RConn1 -- Release Gate/LConn1
  Release Gate/RConn1 -- Output/RConn1
  FIFO Queue/LConn1 -- Input/RConn1

== system Architecture/Router14/Clocked FIFO5 ==
  Event-Based Random Number : EventBasedRandomNumber  Distribution=Gaussian (normal)  meanNorm=E  stdNorm=S
  FIFO Queue : FIFOQueue  Capacity=F  StatNumberInBlock=on
      settings: OutputPortMap=o1
  Release Gate : ReleaseGate  OpenGateUpon=Function call from port fcn
  Time-Based Function-Call Generator : TimeBasedFunctionCallGenerator  EventGenerationMode=Period from port  Period=T
  Input : PMIOPort  Side=Left
  Output : PMIOPort  Port=2  Side=Right
  #n : Outport
  wires:
  Event-Based Random Number/1 -> Time-Based Function-Call Generator/1
  FIFO Queue/1 -> #n/1
  Time-Based Function-Call Generator/1 -> Release Gate/1
  connections:
  FIFO Queue/RConn1 -- Release Gate/LConn1
  Release Gate/RConn1 -- Output/RConn1
  FIFO Queue/LConn1 -- Input/RConn1

== system Architecture/Router15/Attribute Function ==
  MATLAB Function : MATLAB Function  TreatAsAtomicUnit=on
  __DMLF__EDE2FCE__ : EntityDepartureFunctionCallGenerator  TimingFunctionCallF1=Before entity departure  IsInsideAFB=on
  __DMLF__GA__ : GetAttribute  AttributeName=DST|ME  AttributeMissing=Error|Error  AttributeDefaultValue=1|1  AttributeTreatAsVector=1|1  AttributeSendTiming=Before entity departure|Before entity departure  EvaluatedDefaultAttributeValue={ [];[]}  IsInsideAFB=on
      settings: OutputPortMap=o1,o2
  __DMLF__SA__ : SetAttribute  AttributeName=RT  AttributeFrom=Signal port  EvaluatedAttributeValue={ []}  IsInsideAFB=on
  IN : PMIOPort  Side=Left
  OUT : PMIOPort  Port=2  Side=Right
  wires:
  MATLAB Function/1(out_RT) -> __DMLF__SA__/1
  __DMLF__GA__/2 -> MATLAB Function/2(ME)
  __DMLF__GA__/1 -> MATLAB Function/1(DST)
  __DMLF__EDE2FCE__/1 -> MATLAB Function/Trigger
  connections:
  __DMLF__SA__/RConn1 -- OUT/RConn1
  IN/RConn1 -- __DMLF__GA__/LConn1
  __DMLF__GA__/RConn1 -- __DMLF__EDE2FCE__/LConn1
  __DMLF__SA__/LConn1 -- __DMLF__EDE2FCE__/RConn1

== system Architecture/Router15/Clocked FIFO1 ==
  Event-Based Random Number : EventBasedRandomNumber  Distribution=Gaussian (normal)  meanNorm=E  stdNorm=S
  FIFO Queue : FIFOQueue  Capacity=F  StatNumberInBlock=on
      settings: OutputPortMap=o1
  Release Gate : ReleaseGate  OpenGateUpon=Function call from port fcn
  Time-Based Function-Call Generator : TimeBasedFunctionCallGenerator  EventGenerationMode=Period from port  Period=T
  Input : PMIOPort  Side=Left
  Output : PMIOPort  Port=2  Side=Right
  #n : Outport
  wires:
  Event-Based Random Number/1 -> Time-Based Function-Call Generator/1
  FIFO Queue/1 -> #n/1
  Time-Based Function-Call Generator/1 -> Release Gate/1
  connections:
  FIFO Queue/RConn1 -- Release Gate/LConn1
  Release Gate/RConn1 -- Output/RConn1
  FIFO Queue/LConn1 -- Input/RConn1

== system Architecture/Router15/Clocked FIFO2 ==
  Event-Based Random Number : EventBasedRandomNumber  Distribution=Gaussian (normal)  meanNorm=E  stdNorm=S
  FIFO Queue : FIFOQueue  Capacity=F  StatNumberInBlock=on
      settings: OutputPortMap=o1
  Release Gate : ReleaseGate  OpenGateUpon=Function call from port fcn
  Time-Based Function-Call Generator : TimeBasedFunctionCallGenerator  EventGenerationMode=Period from port  Period=T
  Input : PMIOPort  Side=Left
  Output : PMIOPort  Port=2  Side=Right
  #n : Outport
  wires:
  Event-Based Random Number/1 -> Time-Based Function-Call Generator/1
  FIFO Queue/1 -> #n/1
  Time-Based Function-Call Generator/1 -> Release Gate/1
  connections:
  FIFO Queue/RConn1 -- Release Gate/LConn1
  Release Gate/RConn1 -- Output/RConn1
  FIFO Queue/LConn1 -- Input/RConn1

== system Architecture/Router15/Clocked FIFO3 ==
  Event-Based Random Number : EventBasedRandomNumber  Distribution=Gaussian (normal)  meanNorm=E  stdNorm=S
  FIFO Queue : FIFOQueue  Capacity=F  StatNumberInBlock=on
      settings: OutputPortMap=o1
  Release Gate : ReleaseGate  OpenGateUpon=Function call from port fcn
  Time-Based Function-Call Generator : TimeBasedFunctionCallGenerator  EventGenerationMode=Period from port  Period=T
  Input : PMIOPort  Side=Left
  Output : PMIOPort  Port=2  Side=Right
  #n : Outport
  wires:
  Event-Based Random Number/1 -> Time-Based Function-Call Generator/1
  FIFO Queue/1 -> #n/1
  Time-Based Function-Call Generator/1 -> Release Gate/1
  connections:
  FIFO Queue/RConn1 -- Release Gate/LConn1
  Release Gate/RConn1 -- Output/RConn1
  FIFO Queue/LConn1 -- Input/RConn1

== system Architecture/Router15/Clocked FIFO4 ==
  Event-Based Random Number : EventBasedRandomNumber  Distribution=Gaussian (normal)  meanNorm=E  stdNorm=S
  FIFO Queue : FIFOQueue  Capacity=F  StatNumberInBlock=on
      settings: OutputPortMap=o1
  Release Gate : ReleaseGate  OpenGateUpon=Function call from port fcn
  Time-Based Function-Call Generator : TimeBasedFunctionCallGenerator  EventGenerationMode=Period from port  Period=T
  Input : PMIOPort  Side=Left
  Output : PMIOPort  Port=2  Side=Right
  #n : Outport
  wires:
  Event-Based Random Number/1 -> Time-Based Function-Call Generator/1
  FIFO Queue/1 -> #n/1
  Time-Based Function-Call Generator/1 -> Release Gate/1
  connections:
  FIFO Queue/RConn1 -- Release Gate/LConn1
  Release Gate/RConn1 -- Output/RConn1
  FIFO Queue/LConn1 -- Input/RConn1

== system Architecture/Router15/Clocked FIFO5 ==
  Event-Based Random Number : EventBasedRandomNumber  Distribution=Gaussian (normal)  meanNorm=E  stdNorm=S
  FIFO Queue : FIFOQueue  Capacity=F  StatNumberInBlock=on
      settings: OutputPortMap=o1
  Release Gate : ReleaseGate  OpenGateUpon=Function call from port fcn
  Time-Based Function-Call Generator : TimeBasedFunctionCallGenerator  EventGenerationMode=Period from port  Period=T
  Input : PMIOPort  Side=Left
  Output : PMIOPort  Port=2  Side=Right
  #n : Outport
  wires:
  Event-Based Random Number/1 -> Time-Based Function-Call Generator/1
  FIFO Queue/1 -> #n/1
  Time-Based Function-Call Generator/1 -> Release Gate/1
  connections:
  FIFO Queue/RConn1 -- Release Gate/LConn1
  Release Gate/RConn1 -- Output/RConn1
  FIFO Queue/LConn1 -- Input/RConn1

== system Architecture/Router16/Attribute Function ==
  MATLAB Function : MATLAB Function  TreatAsAtomicUnit=on
  __DMLF__EDE2FCE__ : EntityDepartureFunctionCallGenerator  TimingFunctionCallF1=Before entity departure  IsInsideAFB=on
  __DMLF__GA__ : GetAttribute  AttributeName=DST|ME  AttributeMissing=Error|Error  AttributeDefaultValue=1|1  AttributeTreatAsVector=1|1  AttributeSendTiming=Before entity departure|Before entity departure  EvaluatedDefaultAttributeValue={ [];[]}  IsInsideAFB=on
      settings: OutputPortMap=o1,o2
  __DMLF__SA__ : SetAttribute  AttributeName=RT  AttributeFrom=Signal port  EvaluatedAttributeValue={ []}  IsInsideAFB=on
  IN : PMIOPort  Side=Left
  OUT : PMIOPort  Port=2  Side=Right
  wires:
  MATLAB Function/1(out_RT) -> __DMLF__SA__/1
  __DMLF__GA__/2 -> MATLAB Function/2(ME)
  __DMLF__GA__/1 -> MATLAB Function/1(DST)
  __DMLF__EDE2FCE__/1 -> MATLAB Function/Trigger
  connections:
  __DMLF__SA__/RConn1 -- OUT/RConn1
  IN/RConn1 -- __DMLF__GA__/LConn1
  __DMLF__GA__/RConn1 -- __DMLF__EDE2FCE__/LConn1
  __DMLF__SA__/LConn1 -- __DMLF__EDE2FCE__/RConn1

== system Architecture/Router16/Clocked FIFO1 ==
  Event-Based Random Number : EventBasedRandomNumber  Distribution=Gaussian (normal)  meanNorm=E  stdNorm=S
  FIFO Queue : FIFOQueue  Capacity=F  StatNumberInBlock=on
      settings: OutputPortMap=o1
  Release Gate : ReleaseGate  OpenGateUpon=Function call from port fcn
  Time-Based Function-Call Generator : TimeBasedFunctionCallGenerator  EventGenerationMode=Period from port  Period=T
  Input : PMIOPort  Side=Left
  Output : PMIOPort  Port=2  Side=Right
  #n : Outport
  wires:
  Event-Based Random Number/1 -> Time-Based Function-Call Generator/1
  FIFO Queue/1 -> #n/1
  Time-Based Function-Call Generator/1 -> Release Gate/1
  connections:
  FIFO Queue/RConn1 -- Release Gate/LConn1
  Release Gate/RConn1 -- Output/RConn1
  FIFO Queue/LConn1 -- Input/RConn1

== system Architecture/Router16/Clocked FIFO2 ==
  Event-Based Random Number : EventBasedRandomNumber  Distribution=Gaussian (normal)  meanNorm=E  stdNorm=S
  FIFO Queue : FIFOQueue  Capacity=F  StatNumberInBlock=on
      settings: OutputPortMap=o1
  Release Gate : ReleaseGate  OpenGateUpon=Function call from port fcn
  Time-Based Function-Call Generator : TimeBasedFunctionCallGenerator  EventGenerationMode=Period from port  Period=T
  Input : PMIOPort  Side=Left
  Output : PMIOPort  Port=2  Side=Right
  #n : Outport
  wires:
  Event-Based Random Number/1 -> Time-Based Function-Call Generator/1
  FIFO Queue/1 -> #n/1
  Time-Based Function-Call Generator/1 -> Release Gate/1
  connections:
  FIFO Queue/RConn1 -- Release Gate/LConn1
  Release Gate/RConn1 -- Output/RConn1
  FIFO Queue/LConn1 -- Input/RConn1

== system Architecture/Router16/Clocked FIFO3 ==
  Event-Based Random Number : EventBasedRandomNumber  Distribution=Gaussian (normal)  meanNorm=E  stdNorm=S
  FIFO Queue : FIFOQueue  Capacity=F  StatNumberInBlock=on
      settings: OutputPortMap=o1
  Release Gate : ReleaseGate  OpenGateUpon=Function call from port fcn
  Time-Based Function-Call Generator : TimeBasedFunctionCallGenerator  EventGenerationMode=Period from port  Period=T
  Input : PMIOPort  Side=Left
  Output : PMIOPort  Port=2  Side=Right
  #n : Outport
  wires:
  Event-Based Random Number/1 -> Time-Based Function-Call Generator/1
  FIFO Queue/1 -> #n/1
  Time-Based Function-Call Generator/1 -> Release Gate/1
  connections:
  FIFO Queue/RConn1 -- Release Gate/LConn1
  Release Gate/RConn1 -- Output/RConn1
  FIFO Queue/LConn1 -- Input/RConn1

== system Architecture/Router16/Clocked FIFO4 ==
  Event-Based Random Number : EventBasedRandomNumber  Distribution=Gaussian (normal)  meanNorm=E  stdNorm=S
  FIFO Queue : FIFOQueue  Capacity=F  StatNumberInBlock=on
      settings: OutputPortMap=o1
  Release Gate : ReleaseGate  OpenGateUpon=Function call from port fcn
  Time-Based Function-Call Generator : TimeBasedFunctionCallGenerator  EventGenerationMode=Period from port  Period=T
  Input : PMIOPort  Side=Left
  Output : PMIOPort  Port=2  Side=Right
  #n : Outport
  wires:
  Event-Based Random Number/1 -> Time-Based Function-Call Generator/1
  FIFO Queue/1 -> #n/1
  Time-Based Function-Call Generator/1 -> Release Gate/1
  connections:
  FIFO Queue/RConn1 -- Release Gate/LConn1
  Release Gate/RConn1 -- Output/RConn1
  FIFO Queue/LConn1 -- Input/RConn1

== system Architecture/Router16/Clocked FIFO5 ==
  Event-Based Random Number : EventBasedRandomNumber  Distribution=Gaussian (normal)  meanNorm=E  stdNorm=S
  FIFO Queue : FIFOQueue  Capacity=F  StatNumberInBlock=on
      settings: OutputPortMap=o1
  Release Gate : ReleaseGate  OpenGateUpon=Function call from port fcn
  Time-Based Function-Call Generator : TimeBasedFunctionCallGenerator  EventGenerationMode=Period from port  Period=T
  Input : PMIOPort  Side=Left
  Output : PMIOPort  Port=2  Side=Right
  #n : Outport
  wires:
  Event-Based Random Number/1 -> Time-Based Function-Call Generator/1
  FIFO Queue/1 -> #n/1
  Time-Based Function-Call Generator/1 -> Release Gate/1
  connections:
  FIFO Queue/RConn1 -- Release Gate/LConn1
  Release Gate/RConn1 -- Output/RConn1
  FIFO Queue/LConn1 -- Input/RConn1

== system Architecture/Router2/Attribute Function ==
  MATLAB Function : MATLAB Function  TreatAsAtomicUnit=on
  __DMLF__EDE2FCE__ : EntityDepartureFunctionCallGenerator  TimingFunctionCallF1=Before entity departure  IsInsideAFB=on
  __DMLF__GA__ : GetAttribute  AttributeName=DST|ME  AttributeMissing=Error|Error  AttributeDefaultValue=1|1  AttributeTreatAsVector=1|1  AttributeSendTiming=Before entity departure|Before entity departure  EvaluatedDefaultAttributeValue={ [];[]}  IsInsideAFB=on
      settings: OutputPortMap=o1,o2
  __DMLF__SA__ : SetAttribute  AttributeName=RT  AttributeFrom=Signal port  EvaluatedAttributeValue={ []}  IsInsideAFB=on
  IN : PMIOPort  Side=Left
  OUT : PMIOPort  Port=2  Side=Right
  wires:
  MATLAB Function/1(out_RT) -> __DMLF__SA__/1
  __DMLF__GA__/2 -> MATLAB Function/2(ME)
  __DMLF__GA__/1 -> MATLAB Function/1(DST)
  __DMLF__EDE2FCE__/1 -> MATLAB Function/Trigger
  connections:
  __DMLF__SA__/RConn1 -- OUT/RConn1
  IN/RConn1 -- __DMLF__GA__/LConn1
  __DMLF__GA__/RConn1 -- __DMLF__EDE2FCE__/LConn1
  __DMLF__SA__/LConn1 -- __DMLF__EDE2FCE__/RConn1
